simulink model "prach_shortFormat_r2018a"  (Simulink 9.1)
settings: Solver=FixedStepDiscrete  StartTime=0.0  StopTime=prach_short.SimulationTime  FixedStep=1  RelTol=1e-3  EnableMultiTasking=on
PreLoadFcn:
  | warning off Simulink:Commands:SetParamLinkChangeWarn
  | warning off Simulink:Commands:LoadMdlParameterizedLink
  | warning off Simulink:SL_SetParamLinkChangeWarn
  | warning off Simulink:SL_LoadMdlParameterizedLink
  | setup_prach_shortFormat;
InitFcn:
  | setup_prach_shortFormat;
StopFcn:
  | figure;
  | subplot(3,1,1);
  | plot(real(X(:,1))/max(real(X(:,1))),'b');
  | hold on;
  | plot(imag(X(:,1))/max(real(X(:,1))),'r');
  | title('Raw FFT output, matlab reference');
  | subplot(3,1,2);
  | plot(real(PrachOut_DSPBA(1:Nfft))/max(real(PrachOut_DSPBA(1:Nfft))), 'k');
  | hold on;
  | plot(imag(PrachOut_DSPBA(1:Nfft))/max(imag(PrachOut_DSPBA(1:Nfft))), 'm');
  | title('Raw FFT output, DSP Builder');
  | subplot(3,1,3);
  | plot(real(X(:,1))/max(real(X(:,1)))-real(PrachOut_DSPBA(1:Nfft))/max(real(PrachOut_DSPBA(1:Nfft))), 'g');
  | hold on;
  | plot(imag(X(:,1))/max(real(X(:,1)))-imag(PrachOut_DSPBA(1:Nfft))/max(imag(PrachOut_DSPBA(1:Nfft))), 'c');
  | title('Difference');
  | 
  | figure;
  | subplot(2,1,1);
  | plot(real(prach_output(:,1))/max(real(prach_output(:,1))),'b');
  | hold on;
  | plot(imag(prach_output(:,1))/max(real(prach_output(:,1))),'r');
  | title('PRACH output, matlab, normalized ');
  | subplot(2,1,2);
  | for i=1:139
  |     PrachOut139reordered_DSPBA(1+PrachIdxOut139_DSPBA(i)) = PrachOut139_DSPBA(i);
  | end;
  | plot(real(PrachOut139reordered_DSPBA)/max(real(PrachOut139reordered_DSPBA)), 'k');
  | hold on;
  | plot(imag(PrachOut139reordered_DSPBA)/max(imag(PrachOut139reordered_DSPBA)), 'm');
  | title('PRACH output, DSP Builder, normalized');
undefined symbols (not defined in the file or in its folder): BW, dpoly, prach_short, value, waveconfig
libraries: DSPBAPrim x24, DSPBABase x5, DSPBAUtilities x5, simulink x2, PrachLib_FFTshift x1
Description:
  | This design Implements a PRACH detection for short format for TDD configurations.
settings Model: SuppressorTable="22 serialization::archive 17 0 7 0 0 2 2 0 0 0 0 7 0 0 1 0 46 prach_shortFormat_r2018a/Counter Free-Running2 0 7 0 0 2 2 0 0 0 0 7 40 SimulinkFixedPoint:util:Overflowoccurred 0 0 0 7 0  0  0 0 0 0 8 20160523 0 1 0 10 57 55 0 1 41 Simulink:DataType:WarningOverFlowDetected 0 0 0  0  8 20160523 0 10 57 55 0 1 1 0 46 prach_shortFormat_r2018a/Counter Free-Running1 2 2 0 40 SimulinkFixedPoint:util:Overflowoccurred 0 0 0  0  8 20160523 0 10 57 55 0 1 41 Simulink:DataType:WarningOverFlowDetected 0 0 0  0  8 20160523 0 10 57 55 0 1"  Creator=lrigby  LastModifiedBy=5g
settings DataIOCC: LimitDataPoints=on  SignalLoggingSaveFormat=ModelDataLogs
settings OptimizationCC: ExpressionDepthLimit=2147483647  InitFltsAndDblsToZero=on
settings DebuggingCC: SaveWithParameterizedLinksMsg=none  SignalResolutionControl=TryResolveAllWithWarning  SolverPrmCheckMsg=warning  ParameterPrecisionLossMsg=none  StateNameClashWarn=warning
settings HardwareCC: ProdHWDeviceType=ASIC/FPGA  TargetBitPerLong=64  TargetBitPerPointer=64  TargetBitPerSizeT=64  TargetBitPerPtrDiffT=64  TargetLongLongMode=on  TargetIntDivRoundTo=Zero  TargetEndianess=LittleEndian  TargetWordSize=64  TargetHWDeviceType=MATLAB Host  ProdEqTarget=off
settings SFSimCC: SimParseCustomCode=off
settings GRTTargetCC: TargetFcnLib=ansi_tfl_tmw.mat
settings ConfigComp: CovSFcnEnable=off

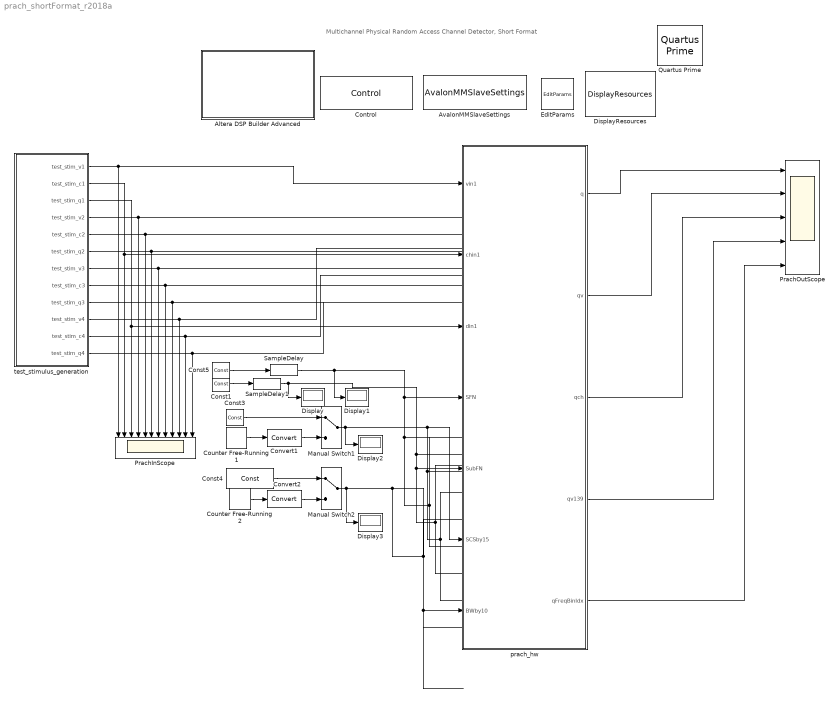
== system prach_shortFormat_r2018a ==
  note: Multichannel Physical Random
      | Access Channel Detector, Short Format
  Altera DSP Builder Advanced : Subsystem  mask(DSP Builder Advanced Blockset Ignored Block){}
      settings: OpenFcn=web('http://www.altera.com', '-new');
      mask Display: image(imread('alteralogo.tif'));
  AvalonMMSlaveSettings : DSPBABase/AvalonMMSlaveSettings
  Const1 : DSPBAPrim/Const  primtype=const  nInputs=0  nOutputs=1  omode=Specify via dialog  otype=uint(8)  scale=2^-0  rndmethod=Unbiased  factor=1  satmethod=Symmetric  shift_vec=[0 1 2 -1]  value=SubF  inPortNames=['+'; '+';]  outPortNames=[' ']  dspbaimage=dspba_prim.svg  text=fprintf('%s', num2str(value));  style=Optimised  visibilities=8 + 1024  floatPrecision=float32_m23  warnSaturation=on  version=20211007  SampleTime=inf
  Const3 : DSPBAPrim/Const  primtype=const  nInputs=0  nOutputs=1  omode=Specify via dialog  otype=uint(2)  scale=1  rndmethod=Unbiased  factor=1  satmethod=Symmetric  shift_vec=[0 1 2 -1]  value=floor(waveconfig.PRACH.Config.SubcarrierSpacing/15)  inPortNames=['+'; '+';]  outPortNames=[' ']  dspbaimage=dspba_prim.svg  text=fprintf('%s', num2str(value));  style=Optimised  visibilities=8 + 1024  floatPrecision=float32_m23  warnSaturation=on  version=20211007  SampleTime=inf
  Const4 : DSPBAPrim/Const  primtype=const  nInputs=0  nOutputs=1  omode=Specify via dialog  otype=uint(4)  scale=1  rndmethod=Unbiased  factor=1  satmethod=Symmetric  shift_vec=[0 1 2 -1]  value=floor(BW/10)  inPortNames=['+'; '+';]  outPortNames=[' ']  dspbaimage=dspba_prim.svg  text=fprintf('%s', num2str(value));  style=Optimised  visibilities=8 + 1024  floatPrecision=float32_m23  warnSaturation=on  version=20211007  SampleTime=inf
  Const5 : DSPBAPrim/Const  primtype=const  nInputs=0  nOutputs=1  omode=Specify via dialog  otype=uint(12)  scale=2^-0  rndmethod=Unbiased  factor=1  satmethod=Symmetric  shift_vec=[0 1 2 -1]  value=SFN  inPortNames=['+'; '+';]  outPortNames=[' ']  dspbaimage=dspba_prim.svg  text=fprintf('%s', num2str(value));  style=Optimised  visibilities=8 + 1024  floatPrecision=float32_m23  warnSaturation=on  version=20211007  SampleTime=inf
  Control : DSPBABase/Control  generate=on  language=VHDL  destination=../rtl  make_full_path=off  path_is_relative=on  autotestbench=on  signaldepth=2  coveragetestbench=off  logs=off  spacewidth=2  spacenum=1  addrwidth=10  datawidth=16  dataendian=Big Endian  hierarchicalnames=on  ramThresholdBits=-1  distRamThresholdBits=-1  mlabThresholdBits=-1  hardMultiplierThresholdLuts=-1  version=20090407  errorOnChanMismatch=1  errorOnGPIOMismatch=0  importModelsimResults=0  cycleAccurate=off  reinterpretCastMult=off  paramFile=prach_shortFormat_r2018a_params.xml
  Convert1 : DSPBAPrim/Convert  primtype=convert  nInputs=1  nOutputs=1  omode=Specify via dialog  otype=uint(2)  scale=1  rndmethod=Biased  factor=1  satmethod=None  shift_vec=[0 1 2 -1]  value=round([0:255]/17)  inPortNames=[' '; ' ';]  outPortNames=[' '; 'c']  dspbaimage=dspba_prim_wide.svg  text=fprintf('convert');  style=Optimised  visibilities=8+64+256+2^17  clipdetect=off  floatPrecision=float32_m23  advOptions=[]  version=20211007
  Convert2 : DSPBAPrim/Convert  primtype=convert  nInputs=1  nOutputs=1  omode=Specify via dialog  otype=uint(8)  scale=1  rndmethod=Biased  factor=1  satmethod=None  shift_vec=[0 1 2 -1]  value=round([0:255]/17)  inPortNames=[' '; ' ';]  outPortNames=[' '; 'c']  dspbaimage=dspba_prim_wide.svg  text=fprintf('convert');  style=Optimised  visibilities=8+64+256+2^17  clipdetect=off  floatPrecision=float32_m23  advOptions=[]  version=20211007
  Counter Free-Running1 : simulink/Sources/Counter Free-Running  NumBits=2  tsamp=-1
  Counter Free-Running2 : simulink/Sources/Counter Free-Running  NumBits=4  tsamp=-1
  Display{,1..3} (4 alike) : Display
  DisplayResources : DSPBAUtilities/DisplayResources  mults=0  luts=0  memorybits=0
  EditParams : DSPBABase/EditParams  version=20090407
  Manual Switch1 : ManualSwitch
  Manual Switch2 : ManualSwitch
  PrachInScope : Scope  NumInputPorts=12
  PrachOutScope : Scope  NumInputPorts=5
  Quartus Prime : DSPBABase/Quartus Prime  version=20090407
  SampleDelay : DSPBAPrim/SampleDelay  primtype=sampdelay  nInputs=1  nOutputs=1  omode=Inherit via internal rule  otype=sfix(16)  scale=2^-15  rndmethod=Unbiased  factor=1  satmethod=Symmetric  shift_vec=[0 1 2 -1]  floatPrecision=float32_m23  value=0  inPortNames=[' '; ' ';]  outPortNames=[' ']  dspbaimage=dspba_prim.svg  text=dpoly(1, eye(1,value+1), 'z')  style=Optimised  visibilities=8 + 1024 + 2^17 + 2^18  flexible=off  slackgroup=0  augmented=0  version=20211007  advOptions=[]
  SampleDelay1 : DSPBAPrim/SampleDelay  primtype=sampdelay  nInputs=1  nOutputs=1  omode=Inherit via internal rule  otype=sfix(16)  scale=2^-15  rndmethod=Unbiased  factor=1  satmethod=Symmetric  shift_vec=[0 1 2 -1]  floatPrecision=float32_m23  value=0  inPortNames=[' '; ' ';]  outPortNames=[' ']  dspbaimage=dspba_prim.svg  text=dpoly(1, eye(1,value+1), 'z')  style=Optimised  visibilities=8 + 1024 + 2^17 + 2^18  flexible=off  slackgroup=0  augmented=0  version=20211007  advOptions=[]
  prach_hw : Subsystem
  test_stimulus_generation : Subsystem
  wires:
  test_stimulus_generation/2(test_stim_c1) -> PrachInScope/2, prach_hw/2(chin1)
  test_stimulus_generation/3(test_stim_q1) -> PrachInScope/3, prach_hw/3(din1)
  test_stimulus_generation/4(test_stim_v2) -> PrachInScope/4
  test_stimulus_generation/5(test_stim_c2) -> PrachInScope/5
  test_stimulus_generation/6(test_stim_q2) -> PrachInScope/6
  test_stimulus_generation/7(test_stim_v3) -> PrachInScope/7
  test_stimulus_generation/8(test_stim_c3) -> PrachInScope/8
  test_stimulus_generation/9(test_stim_q3) -> PrachInScope/9
  test_stimulus_generation/10(test_stim_v4) -> PrachInScope/10
  test_stimulus_generation/11(test_stim_c4) -> PrachInScope/11
  test_stimulus_generation/12(test_stim_q4) -> PrachInScope/12
  test_stimulus_generation/1(test_stim_v1) -> PrachInScope/1, prach_hw/1(vin1)
  Const5/1 -> SampleDelay/1
  Const1/1 -> SampleDelay1/1
  Const3/1 -> Manual Switch1/1
  Const4/1 -> Manual Switch2/1
  Manual Switch1/1 -> prach_hw/6(SCSby15), Display2/1
  Manual Switch2/1 -> prach_hw/7(BWby10), Display3/1
  Counter Free-Running1/1 -> Convert1/1
  Convert1/1 -> Manual Switch1/2
  Counter Free-Running2/1 -> Convert2/1
  Convert2/1 -> Manual Switch2/2
  prach_hw/1(q) -> PrachOutScope/1
  prach_hw/3(qch) -> PrachOutScope/3
  prach_hw/4(qv139) -> PrachOutScope/4
  prach_hw/2(qv) -> PrachOutScope/2
  prach_hw/5(qFreqBinIdx) -> PrachOutScope/5
  SampleDelay/1 -> Display1/1, prach_hw/4(SFN)
  SampleDelay1/1 -> Display/1, prach_hw/5(SubFN)

== system prach_shortFormat_r2018a/Altera DSP Builder Advanced ==

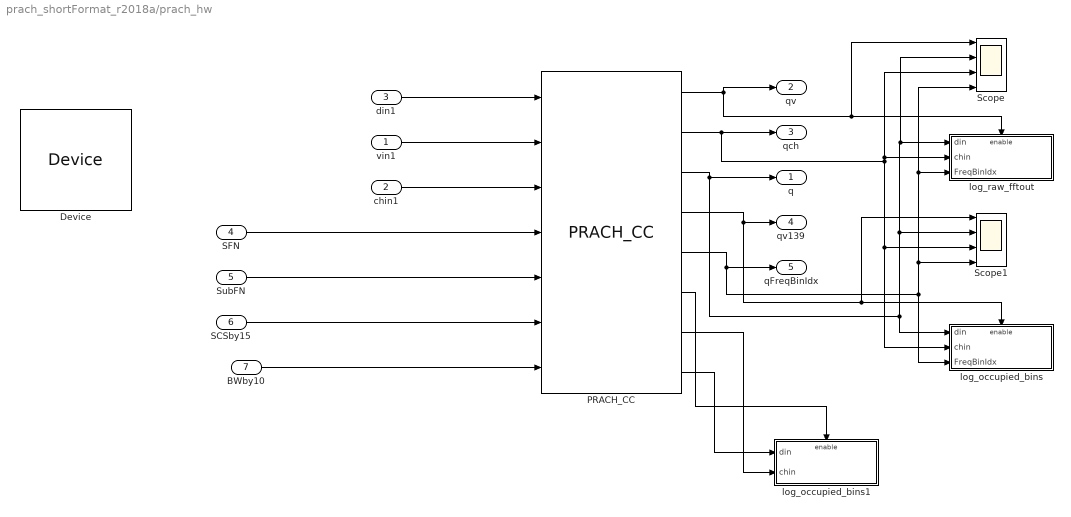
== system prach_shortFormat_r2018a/prach_hw ==
  vin1 : Inport
  chin1 : Inport  Port=2
  din1 : Inport  Port=3
  SFN : Inport  Port=4
  SubFN : Inport  Port=5
  SCSby15 : Inport  Port=6
  BWby10 : Inport  Port=7
  Device : DSPBABase/Device  family=Stratix IV  deviceMember=Stratix IV E  stratix4device=Stratix IV E  hardcopy4device=HardCopy IV E  stratix5device=Stratix V GX  device=AUTO  speed=-3  stratixSpeed=-5  stratix2Speed=-3  stratix3Speed=-3  stratix4gxSpeed=-2  stratix4gtSpeed=-1  cyclone2Speed=-6  cyclone3Speed=-6  arria2Speed=-4  cyclone4eSpeed=-8  stratix5Speed=-3  arria5Speed=-4  arriaSpeed=-6  cyclone3lsSpeed=-7  cyclone5Speed=-6  arria2gzSpeed=-3  nightFurySpeed=-2  ecp2Speed=-7  hardcopycompat=off  version=20140217  max10flashmode=off  max10nomeminit=off
  PRACH_CC : PrachLib_FFTshift/PRACH_CC  InstanceNumber=1
      link override ControlDecode/ChannelOu3t: latency=20
      link override RemoveCP/ChannelOut: latency=2
      link override ScaleAndSelect/ChannelOut: latency=6
      link override ScaleAndSelect/ChannelOut1: latency=14
      link override Stream2BlockConv/ChannelOut: latency=9
      link override VFFT/ChannelOut1: latency=72
  Scope : Scope  NumInputPorts=4
  Scope1 : Scope  NumInputPorts=4
  log_occupied_bins : Subsystem  TreatAsAtomicUnit=on
  log_occupied_bins1 : Subsystem  TreatAsAtomicUnit=on
  log_raw_fftout : Subsystem  TreatAsAtomicUnit=on
  q : Outport  VectorParamsAs1DForOutWhenUnconnected=off
  qv : Outport  Port=2  VectorParamsAs1DForOutWhenUnconnected=off
  qch : Outport  Port=3  VectorParamsAs1DForOutWhenUnconnected=off
  qv139 : Outport  Port=4  VectorParamsAs1DForOutWhenUnconnected=off
  qFreqBinIdx : Outport  Port=5  VectorParamsAs1DForOutWhenUnconnected=off
  wires:
  vin1/1 -> PRACH_CC/2
  chin1/1 -> PRACH_CC/3
  SFN/1 -> PRACH_CC/4
  SubFN/1 -> PRACH_CC/5
  din1/1 -> PRACH_CC/1
  SCSby15/1 -> PRACH_CC/6
  BWby10/1 -> PRACH_CC/7
  PRACH_CC/1 -> qv/1, Scope/1, log_raw_fftout/Enable
  PRACH_CC/2 -> Scope1/3, log_occupied_bins/2(chin), log_raw_fftout/2(chin), Scope/3, qch/1
  PRACH_CC/3 -> q/1, log_occupied_bins/1(din), Scope1/2, Scope/2, log_raw_fftout/1(din)
  PRACH_CC/5 -> Scope1/4, log_raw_fftout/3(FreqBinIdx), Scope/4, log_occupied_bins/3(FreqBinIdx), qFreqBinIdx/1
  PRACH_CC/4 -> qv139/1, Scope1/1, log_occupied_bins/Enable
  PRACH_CC/7 -> log_occupied_bins1/2(chin)
  PRACH_CC/6 -> log_occupied_bins1/Enable
  PRACH_CC/8 -> log_occupied_bins1/1(din)

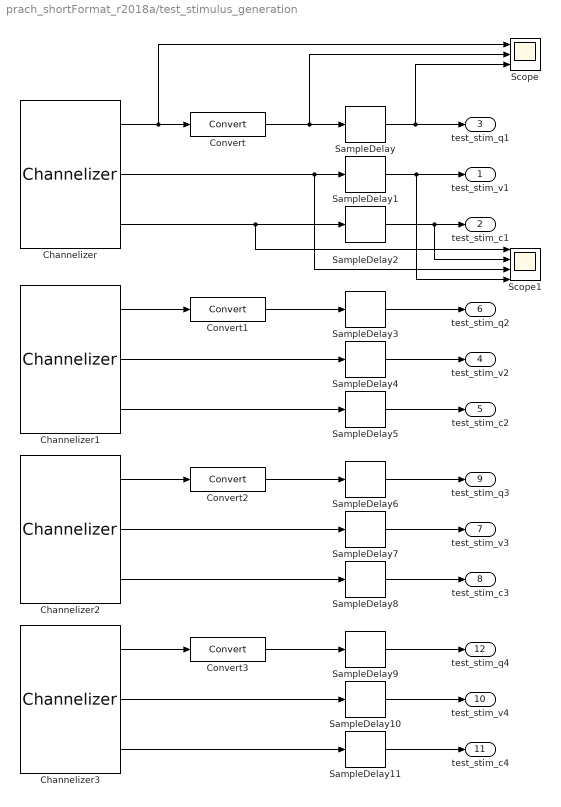
== system prach_shortFormat_r2018a/test_stimulus_generation ==
  Channelizer : DSPBAUtilities/Channelizer  data_input=prach_short.din  folding=prach_short.ClockRate/prach_short.SampleRateMSPS  samples_valid=NTxAnts  samples_idle=0  sample_time=prach_short.SampleTime
  Channelizer1 : DSPBAUtilities/Channelizer  data_input=-prach_short.din  folding=prach_short.ClockRate/prach_short.SampleRateMSPS  samples_valid=NTxAnts  samples_idle=1  sample_time=prach_short.SampleTime
  Channelizer2 : DSPBAUtilities/Channelizer  data_input=prach_short.din  folding=prach_short.ClockRate/prach_short.SampleRateMSPS  samples_valid=NTxAnts  samples_idle=2  sample_time=prach_short.SampleTime
  Channelizer3 : DSPBAUtilities/Channelizer  data_input=-prach_short.din  folding=prach_short.ClockRate/prach_short.SampleRateMSPS  samples_valid=NTxAnts  samples_idle=3  sample_time=prach_short.SampleTime
  Convert{,1..3} (4 alike) : DSPBAPrim/Convert  primtype=convert  nInputs=1  nOutputs=1  omode=Specify via dialog  otype=sfix(16)  scale=2^-15  rndmethod=Biased  factor=1  satmethod=None  shift_vec=[0 1 2 -1]  value=round([0:255]/17)  inPortNames=[' '; ' ';]  outPortNames=[' '; 'c']  dspbaimage=dspba_prim_wide.svg  text=fprintf('convert');  style=Optimised  visibilities=8+64+256+2^17  clipdetect=off  floatPrecision=float32_m23  advOptions=[]  version=20211007
  SampleDelay{,1..6,8..9,11} (10 alike) : DSPBAPrim/SampleDelay  primtype=sampdelay  nInputs=1  nOutputs=1  omode=Inherit via internal rule  otype=sfix(16)  scale=2^-15  rndmethod=Unbiased  factor=1  satmethod=Symmetric  shift_vec=[0 1 2 -1]  floatPrecision=float32_m23  value=0  inPortNames=[' '; ' ';]  outPortNames=[' ']  dspbaimage=dspba_prim.svg  text=dpoly(1, eye(1,value+1), 'z')  style=Optimised  visibilities=8 + 1024 + 2^17 + 2^18  flexible=off  slackgroup=0  augmented=0  version=20211007  advOptions=[]
  SampleDelay10 : DSPBAPrim/SampleDelay  primtype=sampdelay  nInputs=1  nOutputs=1  omode=boolean  otype=sfix(16)  scale=2^-15  rndmethod=Unbiased  factor=1  satmethod=Symmetric  shift_vec=[0 1 2 -1]  floatPrecision=float32_m23  value=0  inPortNames=[' '; ' ';]  outPortNames=[' ']  dspbaimage=dspba_prim.svg  text=dpoly(1, eye(1,value+1), 'z')  style=Optimised  visibilities=8 + 1024 + 2^17 + 2^18  flexible=off  slackgroup=0  augmented=0  version=20211007  advOptions=[]
  SampleDelay7 : DSPBAPrim/SampleDelay  primtype=sampdelay  nInputs=1  nOutputs=1  omode=boolean  otype=sfix(16)  scale=2^-15  rndmethod=Unbiased  factor=1  satmethod=Symmetric  shift_vec=[0 1 2 -1]  floatPrecision=float32_m23  value=0  inPortNames=[' '; ' ';]  outPortNames=[' ']  dspbaimage=dspba_prim.svg  text=dpoly(1, eye(1,value+1), 'z')  style=Optimised  visibilities=8 + 1024 + 2^17 + 2^18  flexible=off  slackgroup=0  augmented=0  version=20211007  advOptions=[]
  Scope : Scope  NumInputPorts=3
  Scope1 : Scope  NumInputPorts=4
  test_stim_v1 : Outport  VectorParamsAs1DForOutWhenUnconnected=off
  test_stim_c1 : Outport  Port=2  VectorParamsAs1DForOutWhenUnconnected=off
  test_stim_q1 : Outport  Port=3  VectorParamsAs1DForOutWhenUnconnected=off
  test_stim_v2 : Outport  Port=4  VectorParamsAs1DForOutWhenUnconnected=off
  test_stim_c2 : Outport  Port=5  VectorParamsAs1DForOutWhenUnconnected=off
  test_stim_q2 : Outport  Port=6  VectorParamsAs1DForOutWhenUnconnected=off
  test_stim_v3 : Outport  Port=7  VectorParamsAs1DForOutWhenUnconnected=off
  test_stim_c3 : Outport  Port=8  VectorParamsAs1DForOutWhenUnconnected=off
  test_stim_q3 : Outport  Port=9  VectorParamsAs1DForOutWhenUnconnected=off
  test_stim_v4 : Outport  Port=10  VectorParamsAs1DForOutWhenUnconnected=off
  test_stim_c4 : Outport  Port=11  VectorParamsAs1DForOutWhenUnconnected=off
  test_stim_q4 : Outport  Port=12  VectorParamsAs1DForOutWhenUnconnected=off
  wires:
  Channelizer/1 -> Scope/1, Convert/1
  Convert/1 -> Scope/2, SampleDelay/1
  SampleDelay/1 -> Scope/3, test_stim_q1/1
  SampleDelay2/1 -> Scope1/2, test_stim_c1/1
  Channelizer/2 -> Scope1/3, SampleDelay1/1
  SampleDelay5/1 -> test_stim_c2/1
  SampleDelay3/1 -> test_stim_q2/1
  Channelizer1/3 -> SampleDelay5/1
  Channelizer1/2 -> SampleDelay4/1
  Convert1/1 -> SampleDelay3/1
  Channelizer1/1 -> Convert1/1
  SampleDelay8/1 -> test_stim_c3/1
  SampleDelay6/1 -> test_stim_q3/1
  Channelizer2/3 -> SampleDelay8/1
  Channelizer2/2 -> SampleDelay7/1
  Convert2/1 -> SampleDelay6/1
  Channelizer2/1 -> Convert2/1
  Channelizer3/2 -> SampleDelay10/1
  SampleDelay9/1 -> test_stim_q4/1
  Convert3/1 -> SampleDelay9/1
  Channelizer3/1 -> Convert3/1
  Channelizer3/3 -> SampleDelay11/1
  SampleDelay11/1 -> test_stim_c4/1
  SampleDelay4/1 -> test_stim_v2/1
  SampleDelay1/1 -> Scope1/4, test_stim_v1/1
  Channelizer/3 -> Scope1/1, SampleDelay2/1
  SampleDelay7/1 -> test_stim_v3/1
  SampleDelay10/1 -> test_stim_v4/1

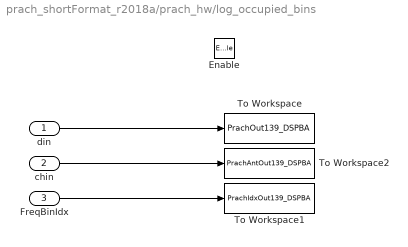
== system prach_shortFormat_r2018a/prach_hw/log_occupied_bins ==
  din : Inport
  chin : Inport  Port=2
  FreqBinIdx : Inport  Port=3
  Enable : EnablePort
  To Workspace : ToWorkspace  VariableName=PrachOut139_DSPBA  SampleTime=-1
  To Workspace1 : ToWorkspace  VariableName=PrachIdxOut139_DSPBA  SampleTime=-1
  To Workspace2 : ToWorkspace  VariableName=PrachAntOut139_DSPBA  SampleTime=-1
  wires:
  chin/1 -> To Workspace2/1
  din/1 -> To Workspace/1
  FreqBinIdx/1 -> To Workspace1/1

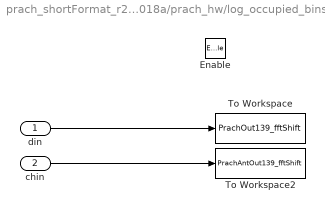
== system prach_shortFormat_r2018a/prach_hw/log_occupied_bins1 ==
  din : Inport
  chin : Inport  Port=2
  Enable : EnablePort
  To Workspace : ToWorkspace  VariableName=PrachOut139_fftShift  SampleTime=-1
  To Workspace2 : ToWorkspace  VariableName=PrachAntOut139_fftShift  SampleTime=-1
  wires:
  din/1 -> To Workspace/1
  chin/1 -> To Workspace2/1

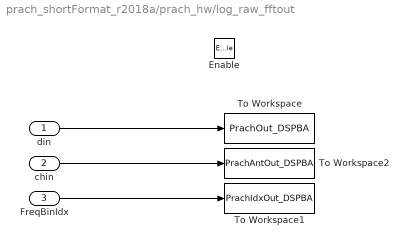
== system prach_shortFormat_r2018a/prach_hw/log_raw_fftout ==
  din : Inport
  chin : Inport  Port=2
  FreqBinIdx : Inport  Port=3
  Enable : EnablePort
  To Workspace : ToWorkspace  VariableName=PrachOut_DSPBA  SampleTime=-1
  To Workspace1 : ToWorkspace  VariableName=PrachIdxOut_DSPBA  SampleTime=-1
  To Workspace2 : ToWorkspace  VariableName=PrachAntOut_DSPBA  SampleTime=-1
  wires:
  FreqBinIdx/1 -> To Workspace1/1
  din/1 -> To Workspace/1
  chin/1 -> To Workspace2/1
